simulink model "ex_6_2_template"  (R2024a)
settings: Solver=VariableStepDiscrete  StartTime=0.0  StopTime=10.0  MaxStep=Ts  RelTol=1e-3
InitFcn:
  | load_data;
values from neighbouring files (symbols this model uses):
  gamma = 0.97    [load_data.m]
settings Model: Creator=puian  LastModifiedBy=puian

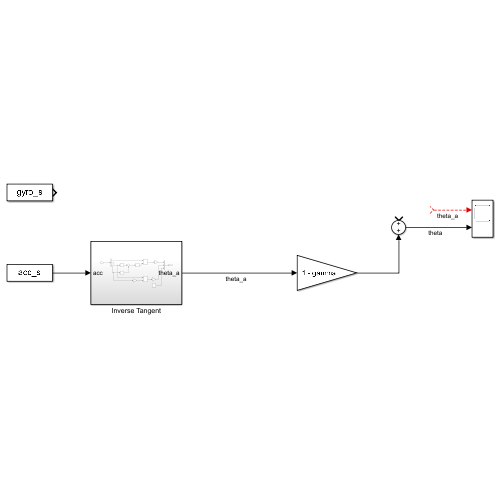
[thumbnail: Simulink's stored preview of the top-level diagram]
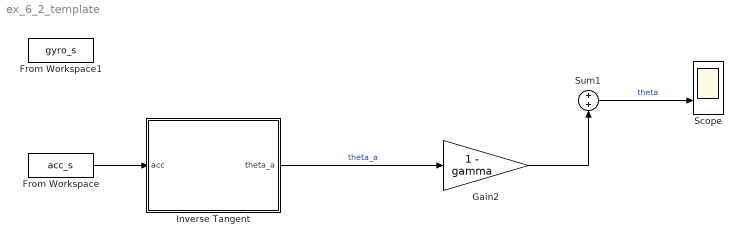
== system ex_6_2_template ==
  From Workspace : FromWorkspace  VariableName=acc_s  Interpolate=off  OutputAfterFinalValue=Holding final value
  From Workspace1 : FromWorkspace  VariableName=gyro_s  Interpolate=off  OutputAfterFinalValue=Holding final value
  Gain2 : Gain  Gain=1 - gamma
  Inverse Tangent : Subsystem
  Scope : Scope  NumInputPorts=2
  Sum1 : Sum  Inputs=+|+
  wires:
  From Workspace/1 -> Inverse Tangent/1(acc)
  Inverse Tangent/1(theta_a) -> Gain2/1  "theta_a"
  Gain2/1 -> Sum1/2
  Sum1/1 -> Scope/2  "theta"
  ? -> Scope/1  "theta_a"

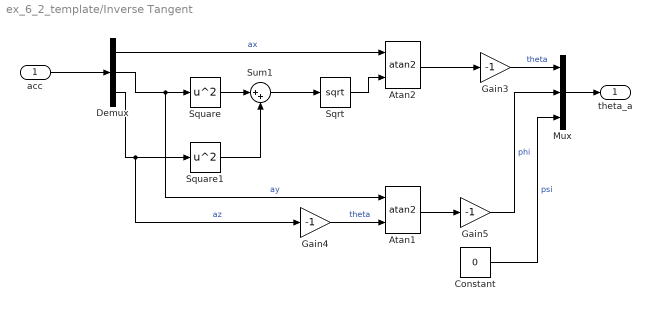
== system ex_6_2_template/Inverse Tangent ==
  acc : Inport
  Atan1 : Trigonometry  Operator=atan2
  Atan2 : Trigonometry  Operator=atan2
  Constant : Constant  Value=0  OutDataTypeStr=single
  Demux : Demux  Outputs=3
  Gain3 : Gain  Gain=-1
  Gain4 : Gain  Gain=-1
  Gain5 : Gain  Gain=-1
  Mux : Mux  Inputs=3
  Sqrt : Sqrt
  Square : Math  Operator=square
  Square1 : Math  Operator=square
  Sum1 : Sum  Inputs=|++
  theta_a : Outport
  wires:
  Demux/3 -> Gain4/1, Square1/1  "az"
  Sqrt/1 -> Atan2/2
  Demux/2 -> Atan1/1, Square/1  "ay"
  Atan1/1 -> Gain5/1
  Gain3/1 -> Mux/1  "theta"
  Gain4/1 -> Atan1/2  "theta"
  Atan2/1 -> Gain3/1
  Square1/1 -> Sum1/2
  Gain5/1 -> Mux/2  "phi"
  Square/1 -> Sum1/1
  Sum1/1 -> Sqrt/1
  Mux/1 -> theta_a/1
  Demux/1 -> Atan2/1  "ax"
  acc/1 -> Demux/1
  Constant/1 -> Mux/3  "psi"
